simulink model "commqpsktx"  (R2013b)
settings: Solver=FixedStepDiscrete  SolverMode=SingleTasking  StartTime=0.0  StopTime=1-0.002  RelTol=1e-3
PreLoadFcn:
  | qpsktxrx = commqpsktxrx_init1();
InitFcn:
  | FrameTime = qpsktxrx.Ts*qpsktxrx.FrameSize*qpsktxrx.Upsampling;
StopFcn:
  | if (strcmp(get_param('commqpsktxrx/Model Parameters','ShowRecvMsg'),'on'))
  |   if exist('received','var')
  |      commqpsktxrx_bits2char;
  |   else
  |      sprintf('%s\n%s\n%s\n%s','Please run the following two lines of code to get the message output:',...
  |       '>> received = <simOut>.get(''received'');',...
  |       '>> commqpsktxrx_bits2char;',...
  |       'where <simOut> is the output of the sim command.')
  |   end
  | end
undefined symbols (not defined in the file or in its folder): dfilt
libraries: dspsigops x5, simulink x4, commdigbbndpm3 x3, commsequence2 x3, dspstat3 x3, dsparch4 x3, commrflib2 x2, commblksprivate x2, dspsrcs4 x2, commutil2 x2, commfilt2 x2, commchan3 x1
(part 2 of 2)

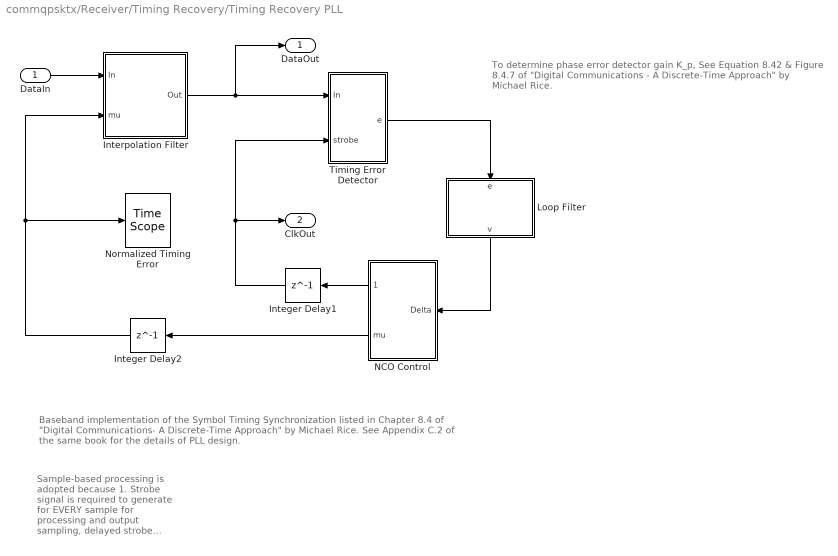
== system commqpsktx/Receiver/Timing Recovery/Timing Recovery PLL ==
  note: Sample-based processing is adopted because
      | 1. Strobe signal is required to generate for EVERY sample for processing and output
      | sampling, delayed strobe signal would affect the accuracy of bit stripping/stuffing
      | 2. The BER performance degrades significantly even with frame size 2 and 4
  note: Baseband implementation of the Symbol Timing Synchronization listed in Chapter 8.4
      | of "Digital Communications- A Discrete-Time Approach" by Michael Rice. See Appendix
      | C.2 of the same book for the details of PLL design.
  note: To determine phase error detector gain K_p, See Equation 8.42 &
      | Figure 8.4.7 of "Digital Communications - A Discrete-Time Approach"
      | by Michael Rice.
  DataIn : Inport
  Integer Delay1 : Delay  DelayLength=1  InputProcessing=Inherited
  Integer Delay2 : Delay  DelayLength=1  InputProcessing=Inherited
  Interpolation Filter : MATLAB Function  TreatAsAtomicUnit=on
  Loop Filter : Subsystem  mask{BnTs=0.01, zeta=1, Kp=qpsktxrx.TimingErrorDetectorGain, K0=qpsktxrx.TimingRecoveryGain, N=qpsktxrx.Upsampling/qpsktxrx.Downsampling}
      mask prompts: BnTs "Loop Bandwidth"; zeta "Loop Damping Factor"; Kp "Phase Detector Gain (Kp)"; K0 "DDS gain (K0)"; N "Number of Samples/symbol (N)"
      mask init:
      | % See C.57 to C.61 in Michael Rice's "Digital Communications 
      | % - A Discrete-Time Approach" for details
      | theta = BnTs/(zeta+0.25/zeta)/N;
      | d = 1 + 2*zeta*theta + theta*theta;
      | K1 = 4*zeta*theta/d;
      | K2 = 4*theta*theta/d;
      | K1 = K1/(Kp*K0);
      | K2 = K2/(Kp*K0);
      mask Display: disp('Loop Filter');
  NCO Control : MATLAB Function
  Normalized Timing Error : TimeScope  DefaultConfigurationName=spbscopes.TimeScopeBlockCfg
      settings: CopyFcn=scopeextensions.ScopeBlock.onCoreBlockCopy(gcbh);  DeleteFcn=scopeextensions.ScopeBlock.callback(gcbh, 'onBlockDelete');  PreSaveFcn=scopeextensions.ScopeBlock.callback(gcbh, 'onModelSave');  NameChangeFcn=scopeextensions.ScopeBlock.callback(gcbh, 'onBlockRename');  DestroyFcn=scopeextensions.ScopeBlock.onBlockDestroy(gcbh)  OpenFcn=scopeextensions.SrcWiredSL.coreBlockCommand('Open',gcbh)  CloseFcn=scopeextensions.ScopeBlock.callback(gcbh, 'onBlockClose');  PreDeleteFcn=scopeextensions.ScopeBlock.callback(gcbh, 'onBlockPreDelete');
  Timing Error Detector : MATLAB Function  TreatAsAtomicUnit=on
  DataOut : Outport
  ClkOut : Outport  Port=2
  wires:
  DataIn/1 -> Interpolation Filter/1(In)
  NCO Control/2(mu) -> Integer Delay2/1
  Integer Delay1/1 -> ClkOut/1, Timing Error Detector/2(strobe)
  NCO Control/1(Underflow) -> Integer Delay1/1
  Interpolation Filter/1(Out) -> DataOut/1, Timing Error Detector/1(In)
  Loop Filter/1(v) -> NCO Control/1(Delta)
  Timing Error Detector/1(e) -> Loop Filter/1(e)
  Integer Delay2/1 -> Interpolation Filter/2(mu), Normalized Timing Error/1

== system commqpsktx/Transmitter/Bit Generation/Barker Code SS ==
  Constant Barker Code : Constant  Value=|  VectorParams1D=off  OutDataTypeStr=double
      | [+1 +1 +1 +1 +1 -1 -1 +1 +1 -1 +1 -1 +1
      | ].' > 0  % Bipolar to Unipolar Conversion
  Out : Outport
  wires:
  Constant Barker Code/1 -> Out/1

== system commqpsktx/Receiver/Data Decoding/Bit Generation/Barker Code SS ==
  Constant Barker Code : Constant  Value=|  VectorParams1D=off  OutDataTypeStr=double
      | [+1 +1 +1 +1 +1 -1 -1 +1 +1 -1 +1 -1 +1
      | ].' > 0  % Bipolar to Unipolar Conversion
  Out : Outport
  wires:
  Constant Barker Code/1 -> Out/1

== system commqpsktx/Receiver/Timing Recovery/Modified Buffer/Modified Buffer ==
  In : Inport
  Enable : EnablePort
  Compare To Constant : simulink/Logic and Bit Operations/Compare To Constant  relop===  const=(bufSize-1)  OutDataTypeStr=boolean  ZeroCross=off
  Counter Limited : simulink/Sources/Counter Limited  uplimit=(bufSize-1)  tsamp=-1
  Delay Line : dspbuff3/Delay Line  siz=bufSize  ic=0  directfeed=on  enable_output=on  hold_output=off  TreatMby1Signals=One channel
  DataOut : Outport
  DataValid : Outport  Port=2
  wires:
  Compare To Constant/1 -> Delay Line/2, DataValid/1
  Delay Line/1 -> DataOut/1
  In/1 -> Delay Line/1
  Counter Limited/1 -> Compare To Constant/1

== system commqpsktx/Receiver/Timing Recovery/Timing Recovery PLL/Loop Filter ==
  note: Proportional-Plus-Integrator Loop Filter,
      | Infinite DC Response to guarantee convergence
  e : Inport
  Digital Filter : dsparch4/Digital Filter  TypePopup=IIR (poles & zeros)  IIRFiltStruct=Direct form II transposed  AllPoleFiltStruct=Direct form  FIRFiltStruct=Direct form  CoeffSource=Specify via dialog  NumCoeffs=[1 0]  DenCoeffs=[1 -1]  BiQuadCoeffs=[1 0.3 0.4 1 0.1 0.2]  LatticeCoeffs=[0.2 0.4]  denIgnore=on  FiltPerSampPopup=One filter per frame  IC=0  ICnum=0  ICden=0  roundingMode=Floor  overflowMode=off  ScaleValues=1  scaleValueFracLength=14  stageInFracLength=15  stageOutFracLength=15  FilterSource=Specify via dialog  dfiltObjectName=dfilt.dffir([1 2 1])  InputProcessing=Columns as channels (frame based)
  K1 : Gain  Gain=K1
  K2 : Gain  Gain=K2
  Sum2 : Sum  SaturateOnIntegerOverflow=on  InputSameDT=on  OutDataTypeStr=Inherit: Same as first input
  v : Outport
  wires:
  K2/1 -> Digital Filter/1
  Digital Filter/1 -> Sum2/2
  Sum2/1 -> v/1
  e/1 -> K2/1, K1/1
  K1/1 -> Sum2/1

== matlab function commqpsktx/Receiver/Timing Recovery/Calculate Number of Valid Samples ==
  data: Clk input; numValid output
function numValid = numValidCalc(Clk)
% Calculate the number of valid outputs in the current received frame. The
% typical value is 100 valid outputs in a 200-element frame. However, in
% bit stuffing case we have 101 valid outputs, and in bit stripping case we 
% have 99 valid outputs.
%
% Input:
%   Clk - Strobe signal
% Output:
%   NumValid - Number of valid outputs in the current received frame 
%#codegen
numValid = sum(Clk~=0);

== matlab function commqpsktx/Receiver/Coarse Frequency Compensation/Find Frequency Offset/Find Frequency Offset ==
  data: N input; FreqOffset output; Tf input; FFTSig input; qpsktxrx parameter
function FreqOffset  = findfreqoffset(N, Tf, FFTSig, qpsktxrx)
% Find frequency offset
% Input:
%   N - Frame size
%   Tf - Two-element vector:  [Frame time, Offset time]
%   FFTSig - Result of FFT
%   M - Modulation alphabet size
% Output:
%   FreqOffset - Estimated frequency offset
%#codegen

M = qpsktxrx.M; 
FFTSize = length(FFTSig);
FFTSig = fftshift(FFTSig);
[~, maxIdx] = max(FFTSig); % Find index of max magnitude
OffsetIdx = maxIdx-1-FFTSize/2; % Convert to index symmetric with 0
Ts = Tf(1)/N; % Sample time
delta_f = 1/Ts/FFTSize; % Frequency resolution of FFT 
FreqOffset = OffsetIdx*delta_f/M;% Map offset index back to frequency

== matlab function commqpsktx/Receiver/Data Decoding/Phase Offset Estimator/Phase Offset Detection ==
  data: In input; Out output
function Out = phasedecision(In)
% Map the estimated phase to one of -pi, -pi/2, 0, pi/2,  
%#codegen
Out = round(In.*2./pi)./2.*pi;
% The above processing is equivalent to the following processing using
% if/else statements
%
% if In<pi/4 && In>-pi/4
%     Out = 0;
% elseif In>=pi/4 && In<pi*3/4
%     Out = pi/2;
% elseif In>=pi*3/4 || In<=-pi*3/4
%     Out = -pi;
% else
%     Out = -pi/2;
% end

== matlab function commqpsktx/Receiver/Fine Frequency Compensation/PED ==
  data: In input; e output
function e = PED(In)
% Implementation of Maximum Likelihood Phase Error Detector listed in
% Chapter 7.2.2 of "Digital Communications - A Discrete-Time Approach" by
% Michael Rice. This employs a decision directed method.
% 
% Input: 
%   In - Input samples, oversampled by two
% Output:
%   e - Phase error, de
%#codegen

e = sign(real(In)).*imag(In) - sign(imag(In)).*real(In);

== matlab function commqpsktx/Receiver/Timing Recovery/Timing Recovery PLL/Interpolation Filter ==
  data: In input; Out output; mu input
function Out = interp_filter(In, mu)
% Prabolic piecewise polynomial interpolator, Farrow Interpolator with 
% alpha = 1/2, see Figure 8.4.16 of "Digital Communications - A 
% Discrete-Time Approach" by Michael Rice.
% Input:
%   In - Input samples, oversampled by two
%   mu - Difference between actual sampling instant and the optimal instant,
%        between zero and one
% Output:
%   Out - Interpolation output
%#codegen
persistent delay1 delay2 delay3; % Input delayed by 1, 2 and 3 samples
if isempty(delay1)
    [delay1, delay2, delay3] = deal(complex(0,0));
end

K = -0.5;

Out = delay2 + mu.*(K.*(In+delay2+delay3)+(1-K).*delay1)...
      + K.*(delay1+delay2-In-delay3).*mu.^2;
  
% Update delay buffers
delay3 = delay2;
delay2 = delay1;
delay1 = In;

== matlab function commqpsktx/Receiver/Timing Recovery/Timing Recovery PLL/NCO Control ==
  data: Delta input; Underflow output; mu output; qpsktxrx parameter
function [Underflow, mu] = NCO_ctrl(Delta, qpsktxrx)
% Implementation of modulo-1 counter for interpolation control listed in
% Figure 8.4.19 of "Digital Communications - A Discrete-Time Approach"
% by Michael Rice. See design details in Chapter 8.4.3 of the same book.
% 
% Input:
%   Delta - Loop filter output. If loop is in lock, delta would be small
%   qpsktxrx - Simulation parameter structure
% Output:
%   Underflow - Indicator of counter underflow. This is the strobe signal
%   for downstream processing
%   mu - Difference between actual sampling instant and the optimal instant,
%        between zero and one
%#codegen

% delay1 - Counter value delayed by 1 sample
% Regtemp - The estimated timing error normalized by half QPSK symbols
persistent delay1 Regtemp;  
if isempty(delay1)
    [delay1, Regtemp] = deal(0);
end
Upsampling = qpsktxrx.Upsampling;
Downsampling = qpsktxrx.Downsampling;
oversampling = Upsampling/Downsampling;

counter = mod(delay1,1)-Delta-1/oversampling; % decrementing counter
if counter < 0
    Underflow = 1;
    Regtemp = mod(delay1,1)/(Delta+1/oversampling);
else
    Underflow = 0;
end

mu = Regtemp;

% Update delay buffer
delay1 = mod(delay1,1)-Delta-1/oversampling;

== matlab function commqpsktx/Receiver/Timing Recovery/Timing Recovery PLL/Timing Error Detector ==
  data: In input; e output; strobe input
function e = TED(In, strobe)
% Zero-Crossing Timing Error Detector. See "Zero-Crossing Timing Error
% Detector" section in Chapter 8.4.1 of "Digital Communications - A
% Discrete-Time Approach" by Michael Rice. For bit stuffing/stripping
% details, see page 490-494 of the same book.
%
% Input: 
%   In - Input samples, interpolation result
%   strobe - Signal to enable timing error calculation
% Output:
%   e - Timing error
%#codegen
persistent delay1 delay2 delayStrobe; % Input delayed by one and 2 samples, and
% Enable signal delayed by one sample
if isempty(delay1)
    [delay1, delay2] = deal(complex(0,0));
    delayStrobe = 0;
end

if strobe==1 && delayStrobe~=strobe
    e = real(delay1) * (sign(real(delay2)) - sign(real(In))) + ...
        imag(delay1) * (sign(imag(delay2)) - sign(imag(In)));
else
    e = 0;
end

if delayStrobe~=strobe
    % Shift contents in delay register
    delay2 = delay1;
    delay1 = In;
elseif strobe==1
    % Two consecutive high strobes
    delay2 = 0; % Stuff missing sample
    delay1 = In; 
end
% If both current and previous enable signals are 0, skip current sample
% and keep the delayed signals unchanged. (Bit stripping)
delayStrobe = strobe;

== matlab function commqpsktx/Receiver/Data Decoding/Align Data ==
  data: Delay input; RxData input; Data output
function Data  = aligndata(Delay, RxData)
% Extract data from the buffered RxData, using the delay to find the frame 
% start
%
% Input:
% Delay - Index of frame start
% RxData - Buffered symbol-spaced data
% Output -
% Data - Data with the Barker code at frame start
%#codegen
Data = RxData(Delay+1:Delay+length(RxData)/2);
